simulink model "w2project3"  (R2020b)
settings: Solver=VariableStepAuto  StartTime=0.0  StopTime=10.0  RelTol=1e-3
settings Model: DataDictionary=w2project3.sldd  OrderedModelArguments=off  Creator=rutvi  LastModifiedBy=rutvi
settings SolverCC: AlgebraicLoopSolver=LineSearch

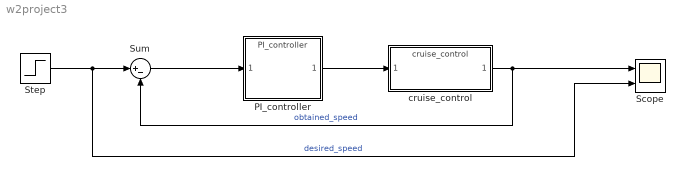
== system w2project3 ==
  PI_controller : ModelReference  ModelNameDialog=PI_controller  SimulationMode=Normal  ModelReferenceVersion=1.7
  Scope : Scope  NumInputPorts=2
  Step : Step  After=u  SampleTime=0
  Sum : Sum  Inputs=|+-
  cruise_control : ModelReference  ModelNameDialog=cruise_control  SimulationMode=Normal  ModelReferenceVersion=1.3
  wires:
  cruise_control/1 -> Scope/1, Sum/2  "obtained_speed"
  Step/1 -> Sum/1, Scope/2  "desired_speed"
  Sum/1 -> PI_controller/1
  PI_controller/1 -> cruise_control/1
